simulink model "Fuel_cell"  (R2020b)
settings: Solver=VariableStepAuto  StartTime=0.0  StopTime=10  RelTol=1e-3
undefined symbols (not defined in the file): DiscIntNeverNeededParam, Ion, Lithium, Pbatt, Ts, Vbatt
libraries: powerlib x17, sdl_lib x8, fl_lib x6, nesl_utility x6, simulink x4, AC6DriveInternalModels x3, simulink_extras x2, electricdrivelib x2, powerlib_extras x1, DC6DriveInternalModels x1
(part 1 of 2)
settings Model: Creator=drim  LastModifiedBy=drim

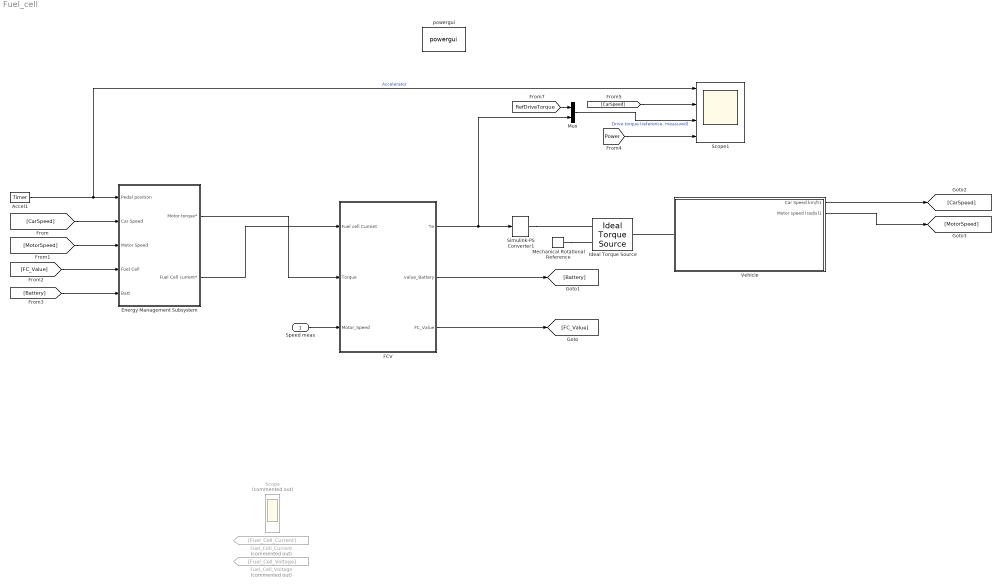
== system Fuel_cell ==
  Speed meas : Inport
  Accel1 : powerlib_extras/Control  Blocks/Timer  t=[0 4 8 12]  e=[0.7 0.25 0.85 -0.7]
      settings: SourceProductBaseCode=PS
  Energy Management Subsystem : Subsystem
      mask init:
      | [X1,X1m,X2,X2m,X3,X4,Y1,Y1m,Y2,Y2m,Y3,Y4,color1,color2]=spsdrivelogo;
      mask Display:
      | patch([X1 X1m],[Y1 Y1m],color1);
      | patch(X3,Y3,color2);
      | plot([X1 X1m X2 X2m X3 X4],[Y1 Y1m Y2 Y2m Y3 Y4]);
  FCV : Subsystem
  Fuel_Cell_Current : Goto  Commented=on  GotoTag=Fuel_Cell_Current
  Fuel_Cell_Voltage : Goto  Commented=on  GotoTag=Fuel_Cell_Voltage
  Ideal Torque Source : fl_lib/Mechanical/Mechanical Sources/Ideal Torque Source
  Mechanical Rotational Reference : fl_lib/Mechanical/Rotational Elements/Mechanical Rotational Reference
  Mux : Mux  Inputs=2
  Scope : Scope  Commented=on  NumInputPorts=3
  Scope1 : Scope  NumInputPorts=4
  Simulink-PS Converter1 : nesl_utility/Simulink-PS Converter  PhysicalDomain=network_engine_domain  SubClassName=ps_input  LeftPortType=input  RightPortType=output  PseudoPeriodic=off  Frequencies=[]  NoiseDistribution=none  NoiseParameters=[]  Unit=1  AffineConversion=off  FilteringAndDerivatives=zero  SimscapeFilterOrder=1  InputFilterTimeConstant=.001  UdotUserProvided=0
  Vehicle : Subsystem
  powergui : powerlib/powergui  Priority=2  SimulationMode=Discrete  SampleTime=Ts  frequency=60  Iterations=50  frequencyindice=0  Pbase=100e6  ErrMax=1e-4  UnitsV=kV  UnitsW=MW  buscounter=0  FunctionMessages=off  echomessages=off  EnableUseOfTLC=off  CurrentSourceSwitches=off  DisableSnubberDevices=off  DisableRonSwitches=off  DisableVfSwitches=off  DisplayEquations=off  AutomaticDiscreteSolvers=off  SolverType=Tustin  Interpol=off  ExternalGateDelay=off  methode=off  Ts=0  x0status=blocks  SPID=off  SwTol=0  HookPort=off  NonlinearTolerance=1e-4  nMaxIteration=100  ContinueOnMaxIteration=off  RestoreLinks=warning  ResistiveCurrentMeasurement=off  Frange=[0:2:500]  Ylog=off  Xlog=on  ShowGrid=off  save=off  variable=ZData  structure=0  ZoomFFT=on  StartTime=0.0  cycles=1  DisplayStyle=1  fundamental=60  FreqAxis=off  MaxFrequency=1000  frequencyindicesteady=1  RmsSteady=1  display=off
  wires:
  Energy Management Subsystem/2(Fuel Cell current*) -> FCV/1(Fuel cell Current)
  Energy Management Subsystem/1(Motor torque*) -> FCV/2("Torque ")
  Speed meas/1 -> FCV/3("Motor_Speed ")
  FCV/1(Te) -> Mux/2, Simulink-PS Converter1/1
  FCV/2(value_Battery) -> [Battery]
  FCV/3(FC_Value) -> [FC_Value]
  Vehicle/1(Car Speed km/h1) -> [CarSpeed]
  Vehicle/2(Motor speed (rad/s)1) -> [MotorSpeed]
  [CarSpeed] -> Energy Management Subsystem/2(Car Speed)
  [MotorSpeed] -> Energy Management Subsystem/3(Motor Speed)
  [FC_Value] -> Energy Management Subsystem/4(Fuel Cell)
  [Battery] -> Energy Management Subsystem/5(Batt)
  Accel1/1 -> Scope1/1, Energy Management Subsystem/1(Pedal position)  "Accelerator"
  [RefDriveTorque] -> Mux/1
  [Power] -> Scope1/4
  Mux/1 -> Scope1/3  "Drive torque (reference, measured)"
  [CarSpeed] -> Scope1/2
  connections:
  Simulink-PS Converter1/RConn1 -- Ideal Torque Source/RConn1
  Mechanical Rotational Reference/LConn1 -- Ideal Torque Source/RConn2
  Vehicle/LConn1 -- Ideal Torque Source/LConn1

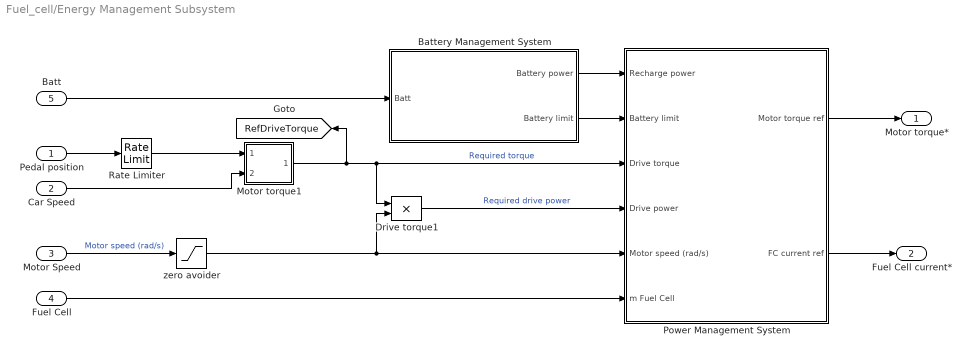
== system Fuel_cell/Energy Management Subsystem ==
  Pedal position : Inport
  Car Speed : Inport  Port=2
  Motor Speed : Inport  Port=3
  Fuel Cell : Inport  Port=4
  Batt : Inport  Port=5
  Battery Management System : Subsystem
      mask init:
      | [X1,X1m,X2,X2m,X3,X4,Y1,Y1m,Y2,Y2m,Y3,Y4,color1,color2]=spsdrivelogo;
      mask Display:
      | patch([X1 X1m],[Y1 Y1m],color1);
      | patch(X3,Y3,color2);
      | plot([X1 X1m X2 X2m X3 X4],[Y1 Y1m Y2 Y2m Y3 Y4]);
  Drive torque1 : Product  Inputs=**  OutDataTypeStr=double
  Motor torque1 : Subsystem
      mask Display: plot([0;1800;2000;2500;3000;3500], [1;1;0.90*1;0.72*1;0.6*1;0.51*1])
  Power Management System : Subsystem
      mask init:
      | [X1,X1m,X2,X2m,X3,X4,Y1,Y1m,Y2,Y2m,Y3,Y4,color1,color2]=spsdrivelogo;
      | power_max = 57000;
      | speed_at_power_max = 5000;
      | speed_max = 6000;
      | [speed,power,torque,p] = drive_enginemodel('MaskGasoline');
      mask Display:
      | patch([X1 X1m],[Y1 Y1m],color1);
      | patch(X3,Y3,color2);
      | plot([X1 X1m X2 X2m X3 X4],[Y1 Y1m Y2 Y2m Y3 Y4]);
  Rate Limiter : RateLimiter  RisingSlewLimit=10  FallingSlewLimit=-10  SampleTimeMode=inherited
  zero avoider : Saturate  UpperLimit=inf  LowerLimit=1
  Motor torque* : Outport
  Fuel Cell current* : Outport  Port=2
  tag scope: RefDriveTorque=global
  wires:
  Motor Speed/1 -> zero avoider/1  "Motor speed (rad/s)"
  Batt/1 -> Battery Management System/1(Batt)
  Pedal position/1 -> Rate Limiter/1
  Fuel Cell/1 -> Power Management System/6(m Fuel Cell)
  Power Management System/1(Motor torque ref) -> Motor torque*/1
  Power Management System/2(FC current ref) -> Fuel Cell current*/1
  Rate Limiter/1 -> Motor torque1/1(Accel)
  Motor torque1/1(torque) -> Drive torque1/1, Power Management System/3(Drive torque), [RefDriveTorque]  "Required torque"
  Drive torque1/1 -> Power Management System/4(Drive power)  "Required drive power"
  Battery Management System/1(Battery power) -> Power Management System/1(Recharge power)
  Car Speed/1 -> Motor torque1/2(N (kmh))
  zero avoider/1 -> Power Management System/5(Motor speed (rad/s)), Drive torque1/2
  Battery Management System/2(Battery limit) -> Power Management System/2(Battery limit)

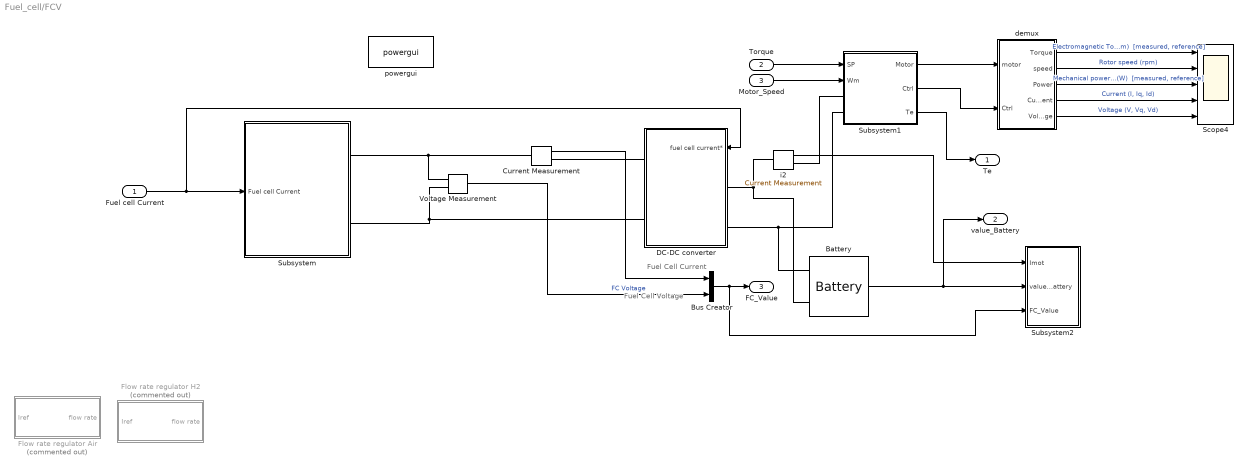
== system Fuel_cell/FCV ==
  note: Fuel Cell Voltage
  note: Fuel Cell Current
  Fuel cell Current : Inport
  "Torque " : Inport  Port=2
  "Motor_Speed " : Inport  Port=3
  Battery : electricdrivelib/Extra Sources/Battery  BatType=Lithium-Ion  ShowTempParam=off  ThermalPreset=no  ShowAgeParam=off  NomV=200  NomQ=5.4  SOC=100  Batt_Tr=30  PresetModel=on  MaxQ=5.4  MinV=150  FullV=232.7974  Dis_rate=2.3478  R=0.37037  Normal_OP=4.8835  expZone="[216.0772     0.2653043]"  current=[6.5 13 32.5]  Units=Time  Tci=20  NomT=20  T2=-30  MaxQ2=4.8  FullV2=7.1  Normal_OP2=5.655  expZone2="[6.58           1]"  Rca=0.6  ti=2000  Dp=0  Neq0=0  Tsim=1e6  Ta1=25  Qeol=5.4*0.9  Reol=0.013333*1.2  Char_age=[2.3478, 3]  Dis_age=[2.3478, 10]  N1=1500  N2=10500  N3=1000  N4=1400  Ta2=45  N5=950
  Bus Creator : BusCreator  Inputs=2
  Current Measurement : powerlib/Measurements/Current Measurement  PhasorSimulation=off  OutputType=Complex  PSBequivalent=0
  DC-DC converter : Subsystem
  Flow rate regulator Air : Subsystem  Commented=on
  Flow rate regulator H2 : Subsystem  Commented=on
  Scope4 : Scope  NumInputPorts=5
  Subsystem : Subsystem
  Subsystem1 : Subsystem
  Subsystem2 : Subsystem
  Voltage Measurement : powerlib/Measurements/Voltage Measurement  PhasorSimulation=off  OutputType=Complex  PSBequivalent=0
  demux : Subsystem
  i2 : powerlib/Measurements/Current Measurement  PhasorSimulation=off  OutputType=Complex  PSBequivalent=0
  powergui : powerlib/powergui  Priority=1  SimulationMode=Discrete  SampleTime=50e-6  frequency=60  Iterations=50  frequencyindice=0  Pbase=100e6  ErrMax=1e-4  UnitsV=kV  UnitsW=MW  buscounter=0  FunctionMessages=off  echomessages=off  EnableUseOfTLC=off  CurrentSourceSwitches=off  DisableSnubberDevices=off  DisableRonSwitches=off  DisableVfSwitches=off  DisplayEquations=off  AutomaticDiscreteSolvers=off  SolverType=Tustin/Backward Euler (TBE)  Interpol=off  ExternalGateDelay=off  methode=off  Ts=100  x0status=blocks  SPID=on  SwTol=0  HookPort=off  NonlinearTolerance=1e-4  nMaxIteration=100  ContinueOnMaxIteration=off  RestoreLinks=warning  ResistiveCurrentMeasurement=off  Frange=[0:2:500]  Ylog=off  Xlog=on  ShowGrid=off  save=off  variable=ZData  structure=0  ZoomFFT=off  StartTime=0.0  cycles=1  DisplayStyle=1  fundamental=60  FreqAxis=off  MaxFrequency=1000  frequencyindicesteady=1  RmsSteady=1  display=off
  Te : Outport
  value_Battery : Outport  Port=2
  FC_Value : Outport  Port=3
  wires:
  Fuel cell Current/1 -> DC-DC converter/1(fuel cell current*), Subsystem/1(Fuel cell Current)
  Bus Creator/1 -> Subsystem2/3(FC_Value), FC_Value/1
  Subsystem1/1(Motor) -> demux/1(motor)
  Battery/1 -> Subsystem2/2(value_Battery), value_Battery/1
  Subsystem1/2(Ctrl) -> demux/2(Ctrl)
  Voltage Measurement/1 -> Bus Creator/2  "FC Voltage"
  "Torque "/1 -> Subsystem1/1(SP)
  Current Measurement/1 -> Bus Creator/1
  "Motor_Speed "/1 -> Subsystem1/2(Wm)
  Subsystem1/3(Te) -> Te/1
  demux/1(Torque) -> Scope4/1  "Electromagnetic Torque (Nm)  [measured, reference]"
  demux/2(speed) -> Scope4/2  "Rotor speed (rpm)"
  demux/3(Power) -> Scope4/3  "Mechanical power (W)  [measured, reference]"
  demux/4(Current) -> Scope4/4  "Current (I, Iq, Id)"
  demux/5(Voltage) -> Scope4/5  "Voltage (V, Vq, Vd)"
  i2/1 -> Subsystem2/1(Imot)
  connections:
  Voltage Measurement/LConn1 -- Current Measurement/LConn1 -- Subsystem/RConn1
  Battery/LConn1 -- i2/LConn1 -- DC-DC converter/LConn1
  Subsystem/RConn2 -- Voltage Measurement/LConn2 -- DC-DC converter/RConn2
  Battery/LConn2 -- Subsystem1/LConn2 -- DC-DC converter/LConn2
  Current Measurement/RConn1 -- DC-DC converter/RConn1
  i2/RConn1 -- Subsystem1/LConn1

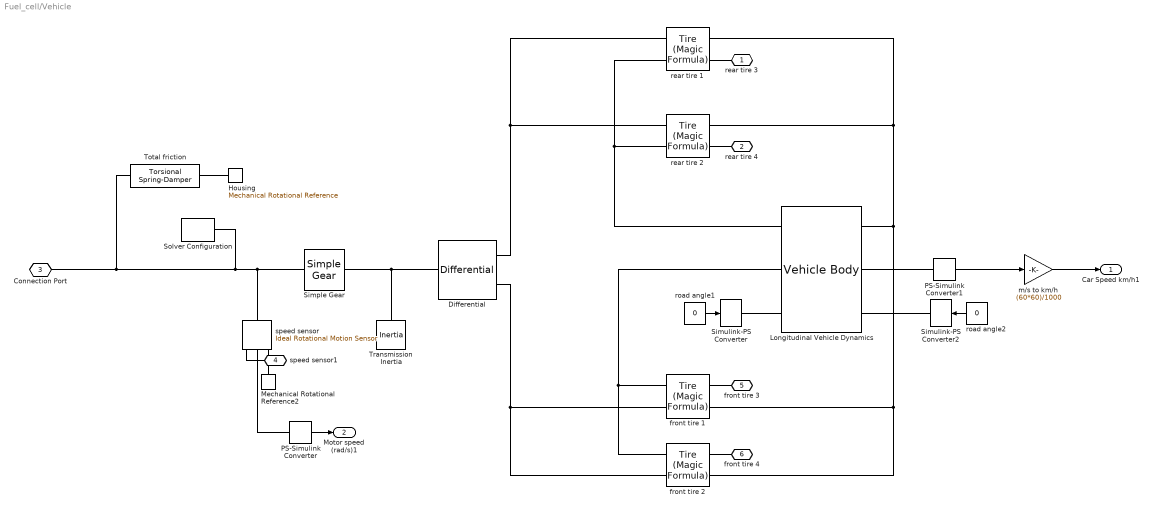
== system Fuel_cell/Vehicle ==
  Differential : sdl_lib/Gears/Differential  driveshaft_location=2  cd_ratio=1  friction_model=1  mu_visc=[ 0 0 ] N*m/(rad/s)  efficiency=[ 0.85 0.92 ]  temperature_TLU=[280, 300, 320] K  efficiency_ss_TLU=[.95, .9, .85]  efficiency_cd_TLU=[.95, .9, .85]  pwr_thr=[.001, .001] W  thermal_mass=50 J/K  T_init=300 K  model_inertia=simscape.enum.onoff.off  carrier_inertia=0.001 kg*m^2  planet_inertia=0.001 kg*m^2
      settings: SourceProductBaseCode=LD
  Housing : fl_lib/Mechanical/Rotational Elements/Mechanical Rotational Reference
  Longitudinal Vehicle Dynamics : sdl_lib/Tires & Vehicles/Vehicle Body  mass=1625 kg  n_w=2  x_f=1.4 m  x_r=1.4 m  y_c=0.5 m  mass_var=simscape.enum.onoff.off  model_pitch=simscape.enum.onoff.off  inertia=4000 kg*m^2  suspension_model=sdl.enum.linearTLU.linear  k_f=1e4 N/m  b_f=1e4 N/(m/s)  k_r=1e4 N/m  b_r=1e4 N/(m/s)  k_f_TLU=[-2000, -1000, 0, 1000, 2000] N  x_f_TLU=[-.4, -.2, 0, .2, .4] m  b_f_TLU=[-200, -100, 0, 100, 200] N  v_f_TLU=[-4, -2, 0, 2, 4] m/s  k_r_TLU=[-2000, -1000, 0, 1000, 2000] N  x_r_TLU=[-.4, -.2, 0, .2, .4] m  b_r_TLU=[-200, -100, 0, 100, 200] N  v_r_TLU=[-4, -2, 0, 2, 4] m/s  interp_method=simscape.enum.interpolation.linear  extrap_method=simscape.enum.extrapolation.linear  model_hardstop=simscape.enum.onoff.off  upper_bound_f=.25 m  lower_bound_f=-.25 m  stop_k_f=1e6 N/m  stop_b_f=150 N/(m/s)  upper_bound_r=.25 m  lower_bound_r=-.25 m  stop_k_r=1e6 N/m  stop_b_r=150 N/(m/s)  initial_pitch=0 rad  initial_pitch_rate=0 rad/s  g=9.81 m/s^2  liftoff_warning=simscape.enum.onoff.off  area=2.711 m^2  Cd=0.26  rho=1.18 kg/m^3  v_specify=on  v_priority=High  v=0 m/s  v_nominal_specify=off  v_nominal_unit=m/s  v_nominal_value=1
  Mechanical Rotational Reference2 : fl_lib/Mechanical/Rotational Elements/Mechanical Rotational Reference
  PS-Simulink Converter : nesl_utility/PS-Simulink Converter  PhysicalDomain=network_engine_domain  SubClassName=ps_output  LeftPortType=input  RightPortType=output  PseudoPeriodic=off  Frequencies=[]  Unit=1  AffineConversion=off
  PS-Simulink Converter1 : nesl_utility/PS-Simulink Converter  PhysicalDomain=network_engine_domain  SubClassName=ps_output  LeftPortType=input  RightPortType=output  PseudoPeriodic=off  Frequencies=[]  Unit=1  AffineConversion=off
  Simple Gear : sdl_lib/Gears/Simple Gear  ratio=7.2  rotation_direction=3-2*(1)  friction_model=1  mu_visc=[ 0 0 ] N*m/(rad/s)  T_noload=0.1 N*m  T_nom=5 N*m  efficiency_nom=0.8  efficiency=0.8  temperature_TLU=[280, 300, 320] K  load_TLU=[1, 5, 10] N*m  efficiency_TLU=[.95, .9, .85]  efficiency_TLU2=[.85, .8, .75; .95, .9, .85; .85, .8, .7]  w_thr=0.01 rad/s  pwr_thr=0.001 W  thermal_mass=50 J/K  enable_faults=simscape.enum.onoff.off  efficiency_fault=0.05  external_fault=simscape.enum.onoff.off  temporal_fault=simscape.enum.onoff.off  fault_time=5 s  fault_angles=pi / 12 rad  report_fault=simscape.enum.assert.action.none  temperature_specify=off  temperature_priority=High  temperature=300 K  temperature_nominal_specify=off  temperature_nominal_unit=K  temperature_nominal_value=1
  Simulink-PS Converter : nesl_utility/Simulink-PS Converter  PhysicalDomain=network_engine_domain  SubClassName=ps_input  LeftPortType=input  RightPortType=output  PseudoPeriodic=off  Frequencies=[]  NoiseDistribution=none  NoiseParameters=[]  Unit=1  AffineConversion=off  FilteringAndDerivatives=zero  SimscapeFilterOrder=1  InputFilterTimeConstant=.001  UdotUserProvided=0
  Simulink-PS Converter2 : nesl_utility/Simulink-PS Converter  PhysicalDomain=network_engine_domain  SubClassName=ps_input  LeftPortType=input  RightPortType=output  PseudoPeriodic=off  Frequencies=[]  NoiseDistribution=none  NoiseParameters=[]  Unit=1  AffineConversion=off  FilteringAndDerivatives=zero  SimscapeFilterOrder=1  InputFilterTimeConstant=.001  UdotUserProvided=0
  Solver Configuration : nesl_utility/Solver Configuration  PhysicalDomain=network_engine_domain  SubClassName=solver  LeftPortType=input  RightPortType=generic  Tones=[]  Harmonics=[]  SimulateNoise=off  Profile=off  UseLocalSampling=off  EnableSwitchedLinearOptims=on  FrequencyDomain=off  UseCCode=off  RelTol=0.001  AbsTol=1e-06  MinStep=1e-09  ToWorkspace=off  RevertToSquareIcSolve=off  NumHomotopyIterations=100  PhasorMode=off  PhasorModeNumHarmonics=1  DoDC=off  ResidualTolerance=1e-5  UseLocalSolver=on  LocalSolverChoice=NE_TRAPEZOIDAL_ADVANCER  LocalSolverSampleTime=Ts  DoFixedCost=off  MaxNonlinIter=3  MaxModeIter=2  ComputeImpulses=off  ImpulseIterations=2  LinearAlgebra=Full  EquationFormulation=NE_TIME_EF  DelaysMemoryBudget=1024  AutomaticFiltering=on  FilteringTimeConstant=0.001  PartitionStorageMethod=AS_NEEDED  PartitionMemoryBudget=1024  PartitionMethod=FAST
  Total friction : sdl_lib/Couplings & Drives/Torsional Spring-Damper  k=0 N*m/rad  mu_visc=0.02 N*m/(rad/s)  trq_coulomb=0 N*m  static_kinetic_ratio=1e9  w_tol=0.001 rad/s  model_hardstop=0  upper_bound=10 deg  lower_bound=-10 deg  k_endstop=1e+6 N*m/rad  D_endstop=10 N*m/(rad/s)  hardstop_model=3  transition=0.001 rad  x0=0 deg
      settings: SourceProductBaseCode=LD  InternalSimscapePortConfiguration="{\"Bottom\":[],\"Left\":[{\"id\":\"R\",\"label\":\"R\",\"type\":\"foundation.mechanical.rotational.rotational\"}],\"Right\":[{\"id\":\"C\",\"label\":\"C\",\"type\":\"foundation.mechanical.rotational.rotational\"}],\"Top\":[]}"
  Transmission Inertia : fl_lib/Mechanical/Rotational Elements/Inertia  inertia=0.5 kg*m^2  num_ports=foundation.enum.numPorts2.one  w_specify=on  w_priority=High  w=0 rad/s  w_nominal_specify=off  w_nominal_unit=rad/s  w_nominal_value=1  t_specify=off  t_priority=High  t=0 N*m  t_nominal_specify=off  t_nominal_unit=N*m  t_nominal_value=1
  front tire 1 : sdl_lib/Tires & Vehicles/Tire (Magic Formula)  parameterization=1  F_z1=3e+3 N  F_x1=3.5e+3 N  kappa1=10  B_m=10  C_m=1.9  D_m=1  E_m=0.97  fz0=4e+3 N  p_Cx=1.685  p_Dx=[ 1.21 -0.037 ]  p_Ex=[ 0.344 0.095 -0.02 0 ]  p_Kx=[ 21.51 -0.163 0.245 ]  p_Hx=[ -0.002 0.002 ]  p_Vx=[ 0 0 ]  v_tr_thr=0.1 m/s  r_e=0.25 m  model_compliance=1  stiffness=1e5 N/m  damping=400 N/(m/s)  model_inertia=1  inertia=0.25 kg*m^2  initial_velocity=0 rad/s  model_resistance=0  resistance_model=1  coeff=0.015  p_tire=250e3 Pa  alpha=-0.003  beta=0.97  coeff_a=84e-4  coeff_b=6.2e-4 s/m  coeff_c=1.6e-4 s^2/m^2  v_thr=1e-3 m/s
  front tire 2 : sdl_lib/Tires & Vehicles/Tire (Magic Formula)  parameterization=1  F_z1=3e+3 N  F_x1=3.5e+3 N  kappa1=10  B_m=10  C_m=1.9  D_m=1  E_m=0.97  fz0=4e+3 N  p_Cx=1.685  p_Dx=[ 1.21 -0.037 ]  p_Ex=[ 0.344 0.095 -0.02 0 ]  p_Kx=[ 21.51 -0.163 0.245 ]  p_Hx=[ -0.002 0.002 ]  p_Vx=[ 0 0 ]  v_tr_thr=0.1 m/s  r_e=0.25 m  model_compliance=1  stiffness=1e5 N/m  damping=400 N/(m/s)  model_inertia=1  inertia=0.25 kg*m^2  initial_velocity=0 rad/s  model_resistance=0  resistance_model=1  coeff=0.015  p_tire=250e3 Pa  alpha=-0.003  beta=0.97  coeff_a=84e-4  coeff_b=6.2e-4 s/m  coeff_c=1.6e-4 s^2/m^2  v_thr=1e-3 m/s
  m/s to km/h : Gain  Gain=(60*60)/1000
  rear tire 1 : sdl_lib/Tires & Vehicles/Tire (Magic Formula)  parameterization=1  F_z1=3e+3 N  F_x1=3.5e+3 N  kappa1=10  B_m=10  C_m=1.9  D_m=1  E_m=0.97  fz0=4e+3 N  p_Cx=1.685  p_Dx=[ 1.21 -0.037 ]  p_Ex=[ 0.344 0.095 -0.02 0 ]  p_Kx=[ 21.51 -0.163 0.245 ]  p_Hx=[ -0.002 0.002 ]  p_Vx=[ 0 0 ]  v_tr_thr=0.1 m/s  r_e=0.25 m  model_compliance=1  stiffness=1e5 N/m  damping=400 N/(m/s)  model_inertia=1  inertia=0.25 kg*m^2  initial_velocity=0 rad/s  model_resistance=0  resistance_model=1  coeff=0.015  p_tire=250e3 Pa  alpha=-0.003  beta=0.97  coeff_a=84e-4  coeff_b=6.2e-4 s/m  coeff_c=1.6e-4 s^2/m^2  v_thr=1e-3 m/s
  rear tire 2 : sdl_lib/Tires & Vehicles/Tire (Magic Formula)  parameterization=1  F_z1=3e+3 N  F_x1=3.5e+3 N  kappa1=10  B_m=10  C_m=1.9  D_m=1  E_m=0.97  fz0=4e+3 N  p_Cx=1.685  p_Dx=[ 1.21 -0.037 ]  p_Ex=[ 0.344 0.095 -0.02 0 ]  p_Kx=[ 21.51 -0.163 0.245 ]  p_Hx=[ -0.002 0.002 ]  p_Vx=[ 0 0 ]  v_tr_thr=0.1 m/s  r_e=0.25 m  model_compliance=1  stiffness=1e5 N/m  damping=400 N/(m/s)  model_inertia=1  inertia=0.25 kg*m^2  initial_velocity=0 rad/s  model_resistance=0  resistance_model=1  coeff=0.015  p_tire=250e3 Pa  alpha=-0.003  beta=0.97  coeff_a=84e-4  coeff_b=6.2e-4 s/m  coeff_c=1.6e-4 s^2/m^2  v_thr=1e-3 m/s
  road angle1 : Constant  Value=0
  road angle2 : Constant  Value=0
  speed sensor : fl_lib/Mechanical/Mechanical Sensors/Ideal Rotational Motion Sensor  wrap_angle=simscape.enum.onoff.off  offset=0 rad
  rear tire 3 : PMIOPort  Side=Right
  rear tire 4 : PMIOPort  Port=2  Side=Right
  Connection Port : PMIOPort  Tag=PMCPort  Port=3  Side=Left
  speed sensor1 : PMIOPort  Port=4  Side=Right
  front tire 3 : PMIOPort  Port=5  Side=Right
  front tire 4 : PMIOPort  Port=6  Side=Right
  Car Speed km/h1 : Outport
  Motor speed (rad/s)1 : Outport  Port=2
  wires:
  m/s to km/h/1 -> Car Speed km/h1/1
  road angle1/1 -> Simulink-PS Converter/1
  PS-Simulink Converter1/1 -> m/s to km/h/1
  road angle2/1 -> Simulink-PS Converter2/1
  PS-Simulink Converter/1 -> Motor speed (rad/s)1/1
  connections:
  Longitudinal Vehicle Dynamics/LConn1 -- front tire 1/RConn2 -- front tire 2/RConn2 -- rear tire 1/RConn2 -- rear tire 2/RConn2
  PS-Simulink Converter1/LConn1 -- Longitudinal Vehicle Dynamics/LConn2
  Simple Gear/RConn1 -- Differential/LConn1 -- Transmission Inertia/LConn1
  front tire 2/LConn2 -- front tire 1/LConn2 -- Differential/RConn1
  Mechanical Rotational Reference2/LConn1 -- speed sensor/RConn1
  Total friction/LConn1 -- Connection Port/RConn1 -- Solver Configuration/RConn1 -- speed sensor/LConn1 -- Simple Gear/LConn1
  front tire 2/LConn1 -- Longitudinal Vehicle Dynamics/RConn2 -- front tire 1/LConn1
  rear tire 1/LConn1 -- Longitudinal Vehicle Dynamics/RConn1 -- rear tire 2/LConn1
  rear tire 1/LConn2 -- rear tire 2/LConn2 -- Differential/RConn2
  speed sensor/RConn3 -- speed sensor1/RConn1
  Simulink-PS Converter/RConn1 -- Longitudinal Vehicle Dynamics/RConn3
  front tire 2/RConn1 -- front tire 4/RConn1
  Simulink-PS Converter2/RConn1 -- Longitudinal Vehicle Dynamics/LConn3
  rear tire 1/RConn1 -- rear tire 3/RConn1
  Housing/LConn1 -- Total friction/RConn1
  PS-Simulink Converter/LConn1 -- speed sensor/RConn2
  front tire 1/RConn1 -- front tire 3/RConn1
  rear tire 2/RConn1 -- rear tire 4/RConn1

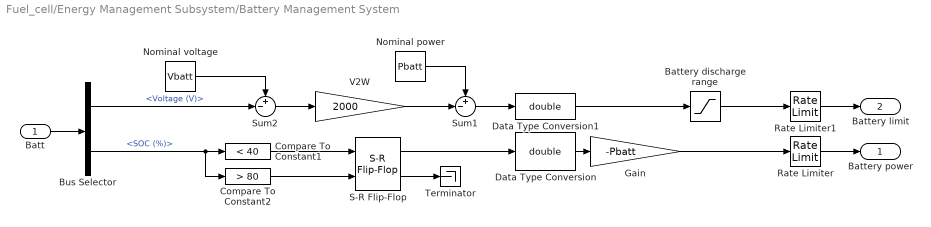
== system Fuel_cell/Energy Management Subsystem/Battery Management System ==
  Batt : Inport
  Battery discharge range : Saturate  UpperLimit=Pbatt  LowerLimit=0
  Bus Selector : BusSelector  OutputSignals=Voltage (V),SOC (%)
  Compare To Constant1 : simulink/Logic and Bit Operations/Compare To Constant  relop=<  const=40  OutDataTypeStr=boolean
  Compare To Constant2 : simulink/Logic and Bit Operations/Compare To Constant  relop=>  const=80  OutDataTypeStr=boolean
  Data Type Conversion : DataTypeConversion  OutDataTypeStr=double  SampleTime=0
  Data Type Conversion1 : DataTypeConversion  OutDataTypeStr=double  SampleTime=0
  Gain : Gain  Gain=-Pbatt
  Nominal power : Constant  Value=Pbatt
  Nominal voltage : Constant  Value=Vbatt
  Rate Limiter : RateLimiter  RisingSlewLimit=Pbatt  FallingSlewLimit=-Pbatt  SampleTimeMode=inherited
  Rate Limiter1 : RateLimiter  RisingSlewLimit=Pbatt*10  FallingSlewLimit=-Pbatt*10  SampleTimeMode=inherited
  S-R Flip-Flop : simulink_extras/Flip Flops/S-R Flip-Flop  initial_condition=0
  Sum1 : Sum  Inputs=+-|
  Sum2 : Sum  Inputs=+-|
  Terminator : Terminator
  V2W : Gain  Gain=2000
  Battery power : Outport
  Battery limit : Outport  Port=2
  wires:
  Batt/1 -> Bus Selector/1
  Gain/1 -> Rate Limiter/1
  S-R Flip-Flop/2 -> Terminator/1
  Bus Selector/2 -> Compare To Constant1/1, Compare To Constant2/1  "<SOC (%)>"
  Data Type Conversion/1 -> Gain/1
  Compare To Constant1/1 -> S-R Flip-Flop/1
  Compare To Constant2/1 -> S-R Flip-Flop/2
  S-R Flip-Flop/1 -> Data Type Conversion/1
  Sum2/1 -> V2W/1
  V2W/1 -> Sum1/2
  Nominal power/1 -> Sum1/1
  Sum1/1 -> Data Type Conversion1/1
  Data Type Conversion1/1 -> Battery discharge range/1
  Battery discharge range/1 -> Rate Limiter1/1
  Bus Selector/1 -> Sum2/2  "<Voltage (V)>"
  Nominal voltage/1 -> Sum2/1
  Rate Limiter1/1 -> Battery limit/1
  Rate Limiter/1 -> Battery power/1

== system Fuel_cell/Energy Management Subsystem/Motor torque1 ==
  Accel : Inport
  N (kmh) : Inport  Port=2
  Abs1 : Abs  SaturateOnIntegerOverflow=on
  Abs2 : Abs  SaturateOnIntegerOverflow=on
  MinMax : MinMax  Inputs=2
  Product : Product  RndMeth=Zero
  Sign : Signum
  Torque vs speed profile : Lookup  InputValues=[0 20 38 60 80 100 120 135 160]  Table=[256 256 256 203 152 122 101 90.5 61]
  rad/s to rpm1 : Gain  Gain=256
  torque : Outport
  wires:
  N (kmh)/1 -> Abs1/1
  Accel/1 -> Abs2/1, Sign/1
  rad/s to rpm1/1 -> MinMax/2
  Torque vs speed profile/1 -> MinMax/1
  Abs1/1 -> Torque vs speed profile/1
  Abs2/1 -> rad/s to rpm1/1
  MinMax/1 -> Product/1
  Sign/1 -> Product/2
  Product/1 -> torque/1

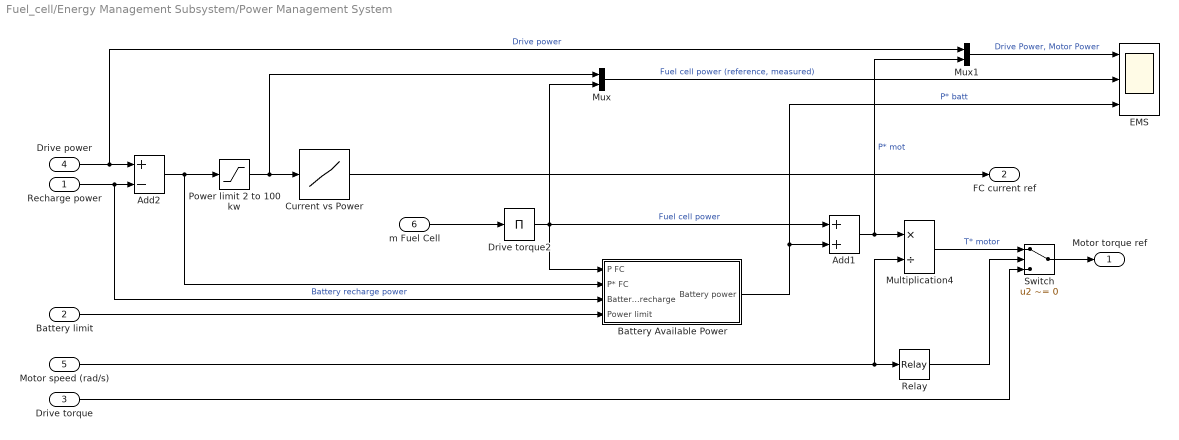
== system Fuel_cell/Energy Management Subsystem/Power Management System ==
  Recharge power : Inport
  Battery limit : Inport  Port=2
  Drive torque : Inport  Port=3
  Drive power : Inport  Port=4
  Motor speed (rad/s) : Inport  Port=5
  m Fuel Cell : Inport  Port=6
  Add1 : Sum
  Add2 : Sum  Inputs=+-
  Battery Available Power : Subsystem
  Current vs Power : Lookup  InputValues=[0,159.95,479.63,795.54,1098.9,1397.7,1691.6,1982,2269.3,2554.2,2837,3117.8,3396.8,3674.2,3950.2,4224.8,4498.1,4770.1,5041,5310.8,5579.6,5847.4,6114.2,6380,6645,6909.1,7172.4,7434.9,7696.5,7957.4,8217.6,8477,8735.7,8993.8,9251.1,9507.8,9763.8,10019,10274,10528,10782,11034,11287,11538,11790,12040,12290,12540,12789,13037,13285,13533,13779,14026,14272,14517,14762,15006,15250,15494,15737,15979,16221,16463,16704,16945,17185,17425,17664,17903,18141,18379,18617,18854,19091,19327,19563,19799,20034,20269,20503,20737,20970,21204,21436,21669,21901,22132,22363,22594,22825,23055,23284,23514,23743,23971,24199,24427,24655,24882,25108,25335,25561,25786,26012,26237,26461,26686,26909,27133,27356,27579,27802,28024,28246,28467,28688,28909,29130,29350,29570,29789,30008,30227,30446,30664,30882,31099,31317,31534,31750,31967,32182,32398,32613,32828,33043,33258,33472,33685,33899,34112,34325,34537,34750,34962,35173,35385,35596,35806,36017,36227,36437,36646,36855,37064,37273,37481,37689,37897,38105,38312,38519,38725,38932,39138,39343,39549,39754,39959,40163,40368,40572,40775,40979,41182,41385,41588,41790,41992,42194,42395,42596,42797,42998,43198,43399,43598,43798,43997,44196,44395,44594,44792,44990,45188,45385,45582,45779,45976,46172,46368,46564,46760,46955,47150,47345,47539,47733,47927,48121,48315,48508,48701,48894,49086,49278,49470,49662,49853,50044,50235,50426,50616,50807,50996,51186,51375,51565,51754,51942,52131,52319,52507,52694,52882,53069,53256,53442,53629,53815,54001,54187,54372,54557,54742,54927,55111,55296,55480,55663,55847,56030,56213,56396,56578,56761,56943,57125,57306,57487,57669,57849,58030,58210,58391,58571,58750,58930,59109,59288,59467,59645,59824,60002,60179,60357,60534,60712,60888,61065,61242,61418,61594,61770,61945,62120,62296,62470,62645,62819,62994,63168,63341,63515,63688,63861,64034,64207,64379,64551,64723,64895,65066,65238,65409,65580,65750,65921,66091,66261,66430,66600,66769,66938,67107,67276,67444,67612,67780,67948,68116,68283,68450,68617,68784,68950,69117,69283,69449,69614,69780,69945,70110,70275,70439,70604,70768,70932,71095,71259,71422,71585,71748,71911,72073,72236,72398,72560,72721,72883,73044,73205,73366,73526,73687,73847,74007,74167,74326,74486,74645,74804,74963,75121,75280,75438,75596,75753,75911,76068,76225,76382,76539,76696,76852,77008,77164,77320,77475,77631,77786,77941,78096,78250,78404,78559,78713,78866,79020,79173,79326,79479,79632,79785,79937,80089,80241,80393,80545,80696,80847,80998,81149,81300,81450,81600,81751,81900,82050,82200,82349,82498,82647,82796,82944,83092,83241,83389,83536,83684,83831,83978,84125,84272,84419,84565,84712,84858,85004,85149,85295,85440,85585,85730,85875,86020,86164,86308,86452,86596,86740,86883,87026,87169,87312,87455,87598,87740,87882,88024,88166,88308,88449,88590,88731,88872,89013,89154,89294,89434,89574,89714,89854,89993,90132,90271,90410,90549,90688,90826,90964,91102,91240,91378,91515,91653,91790,91927,92064,92200,92337,92473,92609,92745,92881,93016,93152,93287,93422,93557,93691,93826,93960,94094,94228,94362,94496,94629,94763,94896,95029,95162,95294,95427,95559,95691,95823,95955,96086,96218,96349,96480,96611,96742,96872,97003,97133,97263,97393,97523,97652,97782,97911,98040,98169,98297,98426,98554,98683,98811,98939,99066,99194,99321,99448,99575,99702,99829,99956,1.0002e+005]  Table=[0,0.39993,1.1997,1.9991,2.7965,3.5871,4.3694,5.1459,5.9178,6.6861,7.4512,8.2135,8.9735,9.7311,10.487,11.241,11.993,12.743,13.492,14.239,14.985,15.73,16.474,17.216,17.957,18.697,19.436,20.174,20.911,21.647,22.382,23.116,23.849,24.581,25.313,26.043,26.773,27.502,28.23,28.958,29.684,30.41,31.136,31.86,32.584,33.307,34.029,34.751,35.472,36.193,36.912,37.632,38.35,39.068,39.785,40.502,41.218,41.934,42.649,43.363,44.077,44.79,45.503,46.215,46.926,47.637,48.348,49.058,49.767,50.476,51.184,51.892,52.599,53.306,54.013,54.718,55.424,56.129,56.833,57.537,58.24,58.943,59.646,60.348,61.049,61.75,62.451,63.151,63.85,64.55,65.248,65.947,66.645,67.342,68.039,68.735,69.432,70.127,70.822,71.517,72.212,72.906,73.599,74.292,74.985,75.677,76.369,77.06,77.751,78.442,79.132,79.822,80.511,81.2,81.889,82.577,83.265,83.952,84.639,85.326,86.012,86.698,87.383,88.068,88.753,89.437,90.121,90.805,91.488,92.17,92.853,93.535,94.216,94.898,95.578,96.259,96.939,97.619,98.298,98.977,99.656,100.33,101.01,101.69,102.37,103.04,103.72,104.4,105.07,105.75,106.42,107.1,107.77,108.45,109.12,109.79,110.47,111.14,111.81,112.48,113.15,113.82,114.5,115.17,115.84,116.51,117.18,117.84,118.51,119.18,119.85,120.52,121.18,121.85,122.52,123.19,123.85,124.52,125.18,125.85,126.51,127.18,127.84,128.5,129.17,129.83,130.49,131.16,131.82,132.48,133.14,133.8,134.46,135.12,135.78,136.44,137.1,137.76,138.42,139.08,139.74,140.4,141.05,141.71,142.37,143.03,143.68,144.34,144.99,145.65,146.3,146.96,147.61,148.27,148.92,149.58,150.23,150.88,151.53,152.19,152.84,153.49,154.14,154.79,155.44,156.09,156.74,157.39,158.04,158.69,159.34,159.99,160.64,161.29,161.94,162.58,163.23,163.88,164.52,165.17,165.82,166.46,167.11,167.75,168.4,169.04,169.69,170.33,170.97,171.62,172.26,172.9,173.55,174.19,174.83,175.47,176.11,176.75,177.39,178.03,178.67,179.31,179.95,180.59,181.23,181.87,182.51,183.15,183.78,184.42,185.06,185.7,186.33,186.97,187.61,188.24,188.88,189.51,190.15,190.78,191.42,192.05,192.68,193.32,193.95,194.58,195.22,195.85,196.48,197.11,197.75,198.38,199.01,199.64,200.27,200.9,201.53,202.16,202.79,203.42,204.05,204.67,205.3,205.93,206.56,207.19,207.81,208.44,209.07,209.69,210.32,210.94,211.57,212.2,212.82,213.45,214.07,214.69,215.32,215.94,216.56,217.19,217.81,218.43,219.06,219.68,220.3,220.92,221.54,222.16,222.78,223.4,224.02,224.64,225.26,225.88,226.5,227.12,227.74,228.36,228.98,229.59,230.21,230.83,231.45,232.06,232.68,233.29,233.91,234.53,235.14,235.76,236.37,236.99,237.6,238.21,238.83,239.44,240.06,240.67,241.28,241.89,242.51,243.12,243.73,244.34,244.95,245.56,246.17,246.78,247.39,248,248.61,249.22,249.83,250.44,251.05,251.66,252.27,252.87,253.48,254.09,254.7,255.3,255.91,256.52,257.12,257.73,258.33,258.94,259.54,260.15,260.75,261.36,261.96,262.57,263.17,263.77,264.38,264.98,265.58,266.18,266.79,267.39,267.99,268.59,269.19,269.79,270.39,270.99,271.59,272.19,272.79,273.39,273.99,274.59,275.19,275.79,276.38,276.98,277.58,278.18,278.77,279.37,279.97,280.56,281.16,281.76,282.35,282.95,283.54,284.14,284.73,285.33,285.92,286.51,287.11,287.7,288.29,288.89,289.48,290.07,290.66,291.26,291.85,292.44,293.03,293.62,294.21,294.8,295.39,295.98,296.57,297.16,297.75,298.34,298.93,299.52,300.11,300.69,301.28,301.87,302.46,303.04,303.63,304.22,304.8,305.39,305.98,306.56,307.15,307.73,308.32,308.9,309.49,310.07,310.65,311.24,311.82,312.41,312.99,313.57,314.15,314.74,315.32,315.9,316.48,317.06,317.64,318.23,318.81,319.39,319.97,320.55,321.13,321.71,322.29,322.86,323.44,324.02,324.6,325.18,325.76,326.33,326.91,327.49,328.07,328.64,329.22,329.79,330.37,330.95,331.52,332.1,332.67,333.25,333.82,334.4,334.97,335.54,336.12,336.69,337.26,337.84,338.41,338.98,339.56,340.13,340.7,341.27,341.84,342.41,342.98,343.56,344.13,344.7,345.27,345.84,346.41,346.98,347.54]
  Drive torque2 : Product  Inputs=*  OutDataTypeStr=double
  EMS : Scope  NumInputPorts=3
  Multiplication4 : Product  Inputs=*/
  Mux : Mux  Inputs=2
  Mux1 : Mux  Inputs=2
  Power limit 2 to 100 kw : Saturate  UpperLimit=100e3  LowerLimit=2e3
  Relay : Relay  OnSwitchValue=300/30*pi  OffSwitchValue=200/30*pi
  Switch : Switch  Criteria=u2 ~= 0
  Motor torque ref : Outport
  FC current ref : Outport  Port=2
  wires:
  Motor speed (rad/s)/1 -> Relay/1, Multiplication4/2
  Drive torque2/1 -> Add1/1, Mux/2, Battery Available Power/1(P FC)  "Fuel cell power"
  Add1/1 -> Multiplication4/1, Mux1/2  "P* mot"
  Drive power/1 -> Add2/1, Mux1/1  "Drive power"
  Add2/1 -> Power limit 2 to 100 kw/1, Battery Available Power/2(P* FC)
  Battery Available Power/1(Battery power) -> Add1/2, EMS/3  "P* batt"
  Current vs Power/1 -> FC current ref/1
  Recharge power/1 -> Add2/2, Battery Available Power/3(Battery recharge)  "Battery recharge power"
  Battery limit/1 -> Battery Available Power/4(Power limit)
  m Fuel Cell/1 -> Drive torque2/1
  Mux/1 -> EMS/2  "Fuel cell power (reference, measured)"
  Power limit 2 to 100 kw/1 -> Current vs Power/1, Mux/1
  Relay/1 -> Switch/2
  Multiplication4/1 -> Switch/1  "T* motor"
  Switch/1 -> Motor torque ref/1
  Drive torque/1 -> Switch/3
  Mux1/1 -> EMS/1  "Drive Power, Motor Power"

== system Fuel_cell/FCV/DC-DC converter ==
  fuel cell current* : Inport
  Bus DC controller : Subsystem
  DC/DC converter : Subsystem
  +Vfc : PMIOPort  Tag=PMCPort  Side=Right
  - Vfc : PMIOPort  Tag=PMCPort  Port=2  Side=Right
  + Vdc : PMIOPort  Tag=PMCPort  Port=3  Side=Left
  - Vdc : PMIOPort  Tag=PMCPort  Port=4  Side=Left
  wires:
  DC/DC converter/1(ifc) -> Bus DC controller/2(ifc)
  Bus DC controller/1(Duty cycle) -> DC/DC converter/1(Duty Cycle)
  fuel cell current*/1 -> Bus DC controller/1(iref)
  connections:
  + Vdc/RConn1 -- DC/DC converter/RConn1
  +Vfc/RConn1 -- DC/DC converter/LConn1
  - Vfc/RConn1 -- DC/DC converter/LConn2
  - Vdc/RConn1 -- DC/DC converter/RConn2

== system Fuel_cell/FCV/Flow rate regulator Air ==
  Iref : Inport
  Compressor response : TransferFcn  Denominator=[1/3 1]
  Fcn1 : Fcn  Expr=60000*8.3145*(273+95)*400*u(1)/(4*96485*(3*101325)*0.5057*.21)
  Saturation : Saturate  UpperLimit=inf  LowerLimit=60
  flow rate : Outport
  wires:
  Iref/1 -> Fcn1/1
  Saturation/1 -> flow rate/1
  Fcn1/1 -> Compressor response/1
  Compressor response/1 -> Saturation/1

== system Fuel_cell/FCV/Flow rate regulator H2 ==
  Iref : Inport
  Fcn1 : Fcn  Expr=60000*8.3145*(273+95)*400*u(1)/(2*96485*(3*101325)*0.919*.9995)
  Saturation : Saturate  UpperLimit=inf  LowerLimit=1
  flow rate : Outport
  wires:
  Fcn1/1 -> Saturation/1
  Saturation/1 -> flow rate/1
  Iref/1 -> Fcn1/1

== system Fuel_cell/FCV/Subsystem ==
  Fuel cell Current : Inport
  Bus Selector : BusSelector  OutputSignals=Current
  Fcn1 : Fcn  Expr=60000*8.3145*(273+95)*400*u(1)/(2*96485*(3*101325)*0.919*.9995)
  Fcn2 : Fcn  Expr=60000*8.3145*(273+95)*400*u(1)/(4*96485*(3*101325)*0.5057*.21)
  Fuel Cell Stack : electricdrivelib/Extra Sources/Fuel Cell Stack  PresetModel=PEMFC - 6 kW - 45 Vdc  FcType=Proton Exchange Membrane (PEM)  Detailed=Detailed  Eoc=[65,63]  NomVI=[133.3,45]  EndVI=[225,37]  Nc=65  n=55  TOp=65  AirFr=300  SuppPress=[1.5,1]  Comp=[99.95,21,1]  SignX=off  SignY=off  FlowRateH2=on  FlowRateAir=on  SystemTemp=off  SystemPH2=off  SystemPAir=off  FCDyn=on  FC_tau=2  Peak_O2=80  V_Under=10
      settings: SourceProductBaseCode=PS
  MinMax : MinMax  Function=max  Inputs=2
  +Vfc : PMIOPort  Side=Right
  -Vfc : PMIOPort  Port=2  Side=Right
  wires:
  MinMax/1 -> Fcn2/1, Fcn1/1
  Bus Selector/1 -> MinMax/1  "<Current>"
  Fuel cell Current/1 -> MinMax/2
  Fcn1/1 -> Fuel Cell Stack/1
  Fcn2/1 -> Fuel Cell Stack/2
  Fuel Cell Stack/1 -> Bus Selector/1
  connections:
  +Vfc/RConn1 -- Fuel Cell Stack/RConn1
  -Vfc/RConn1 -- Fuel Cell Stack/RConn2

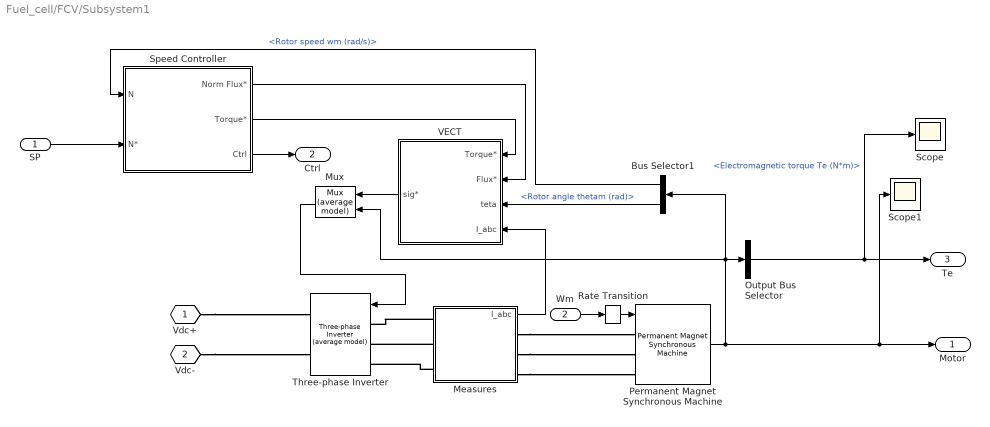
== system Fuel_cell/FCV/Subsystem1 ==
  SP : Inport
  Wm : Inport  Port=2
  Bus Selector1 : BusSelector  OutputSignals=Rotor speed wm (rad/s),Rotor angle thetam (rad)
  Measures : Subsystem
  Mux : AC6DriveInternalModels/Mux (average model)  SystemSampleTime=-1  VariantActivationTime=update diagram  Latency=0  AutoFrameSizeCalculation=off
      settings: SourceProductBaseCode=PS
  Output Bus Selector : BusSelector  OutputSignals=Electromagnetic torque Te (N*m)
  Permanent Magnet Synchronous Machine : powerlib/Machines/Permanent Magnet Synchronous Machine  NbPhases=3  FluxDistribution=Sinusoidal  RotorType=Salient-pole  MechanicalLoad=Speed w  PresetModel=No  ShowDetailedParameters=on  MeasurementBus=off  Resistance=18.7  Inductance=0  dqInductances=[0.02547 0.02816]  La=0.000835  MachineConstant=Flux linkage established by magnets (V.s)  Flux=0.1716  VoltageCst=62.2496  TorqueCst=0.5148  Flat=0  Mechanical=[2.26e-05 1.349e-05 2 0]  PolePairs=2  InitialConditions=[0,0, 0,0]  InitialConditions5ph=[0 0 0 0 0 0]  RefAngle=90 degrees behind phase A axis (modified Park)  IterativeDiscreteModel=Trapezoidal non iterative  TsBlock=-1  TsPowergui=0
      settings: AttributesFormatString=\n
  Rate Transition : RateTransition  OutPortSampleTime=Ts
  Scope : Scope
  Scope1 : Scope
  Speed Controller : Subsystem  mask(Speed controller){SwK=Torque regulation, ramp=[-1000,1000]*10, kp=5, ki=100, fc=100, ctrl_sat=[-256 256], Tsc=120e-6}
      mask prompts: SwK "Regulation type"; ramp "Speed reference ramp (rpm/s) [deceleration,acceleration]"; kp "Proportional gain"; ki "Integral gain"; fc "Speed measurement - low-pass filter cutoff frequency (Hz)"; ctrl_sat "Controller output torque saturation (N.m) [negative,positive]"; Tsc "Controller sampling time (s)"
      mask help: This block implements a PI speed regulator.
      mask init:
      | [X1,X1m,X2,X2m,X3,X4,Y1,Y1m,Y2,Y2m,Y3,Y4,color1,color2]=spsdrivelogo;
      | if SwK == 1
      |     set_param(gcb,'MaskVisibilities',{'on','on','on','on','on','on','on'})
      | else
      |     set_param(gcb,'MaskVisibilities',{'on','off','off','off','off','on','on'})
      | end
      mask TypeOptions SwK: Speed regulation | Torque regulation
      mask Display:
      | patch([X1 X1m],[Y1 Y1m],color1);
      | patch(X3,Y3,color2);
      | plot([X1 X1m X2 X2m X3 X4],[Y1 Y1m Y2 Y2m Y3 Y4]);
  Three-phase Inverter : AC6DriveInternalModels/Three-phase Inverter (average model)  Arms=3  SnubberResistance=5000  SnubberCapacitance=inf  Device=IGBT / Diodes  Ron=1e-3  Lon=0  ForwardVoltages=[0.8,0.8]  ForwardVoltage=0  GTOparameters=[0,0]  IGBTparameters=[1e-6,2e-6]  Measurements=All voltages and currents  converterType=Inverter  SourceFrequency=60  dqInductances="[0.00017415845761   0.00029268882377]"  Flux=0.07111510954334  Resistance=0.0083  p=4
      settings: SourceProductBaseCode=PS
  VECT : Subsystem  mask(VECT){nb_p=4, dqInductances=[0.00017415845761   0.00029268882377], lambda=0.07111510954334, freq_max=20e3, Ts_vect=60e-6, h=0.1}
      mask prompts: nb_p "Motor pairs of poles"; dqInductances "Inductances [ Ld(H) Lq(H) ]:"; lambda "Flux induced by magnets (Wb)"; freq_max "Maximum switching frequency (Hz)"; Ts_vect "Sampling time (s)"; h "Current hysteresis bandwidth (A)"
      mask help: This block implements a vector controller.
      mask init:
      | [X1,X1m,X2,X2m,X3,X4,Y1,Y1m,Y2,Y2m,Y3,Y4,color1,color2]=spsdrivelogo;
      | ib = lambda/(dqInductances(2)-dqInductances(1));
      | Teb = 3/2*nb_p*lambda*ib;
      mask Display:
      | patch([X1 X1m],[Y1 Y1m],color1);
      | patch(X3,Y3,color2);
      | plot([X1 X1m X2 X2m X3 X4],[Y1 Y1m Y2 Y2m Y3 Y4]);
  Vdc+ : PMIOPort  Tag=PMCPort  Side=Left
  Vdc- : PMIOPort  Tag=PMCPort  Port=2  Side=Left
  Motor : Outport
  Ctrl : Outport  Port=2
  Te : Outport  Port=3
  wires:
  Bus Selector1/2 -> VECT/3(teta)  "<Rotor angle thetam (rad)>"
  Speed Controller/3(Ctrl) -> Ctrl/1
  Output Bus Selector/1 -> Scope/1, Te/1  "<Electromagnetic torque Te (N*m)>"
  Mux/1 -> Three-phase Inverter/1
  Rate Transition/1 -> Permanent Magnet Synchronous Machine/1
  SP/1 -> Speed Controller/2(N*)
  Wm/1 -> Rate Transition/1
  VECT/1(sig*) -> Mux/1
  Speed Controller/1(Norm Flux*) -> VECT/2(Flux*)
  Speed Controller/2(Torque*) -> VECT/1(Torque*)
  Permanent Magnet Synchronous Machine/1 -> Scope1/1, Motor/1, Mux/2, Output Bus Selector/1, Bus Selector1/1
  Measures/1(I_abc) -> VECT/4(I_abc)
  Bus Selector1/1 -> Speed Controller/1(N)  "<Rotor speed wm (rad/s)>"
  connections:
  Vdc-/RConn1 -- Three-phase Inverter/RConn2
  Measures/LConn2 -- Three-phase Inverter/LConn2
  Vdc+/RConn1 -- Three-phase Inverter/RConn1
  Measures/RConn2 -- Permanent Magnet Synchronous Machine/LConn2
  Measures/LConn3 -- Three-phase Inverter/LConn3
  Measures/RConn1 -- Permanent Magnet Synchronous Machine/LConn1
  Measures/RConn3 -- Permanent Magnet Synchronous Machine/LConn3
  Measures/LConn1 -- Three-phase Inverter/LConn1

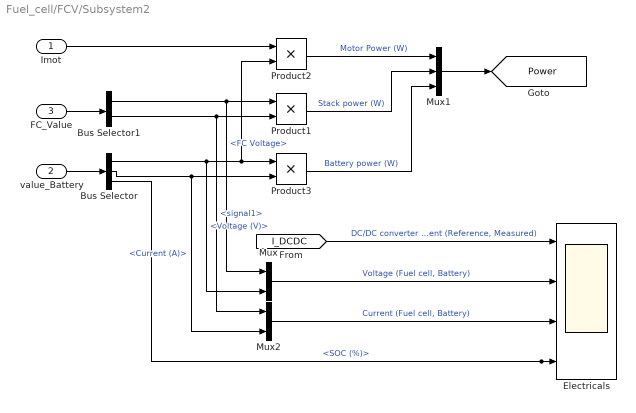
== system Fuel_cell/FCV/Subsystem2 ==
  Imot : Inport
  value_Battery : Inport  Port=2
  FC_Value : Inport  Port=3
  Bus Selector : BusSelector  OutputSignals=Voltage (V),Current (A),SOC (%)
  Bus Selector1 : BusSelector  OutputSignals=FC Voltage,signal1
  Electricals : Scope  NumInputPorts=4
  Mux : Mux  Inputs=2
  Mux1 : Mux  Inputs=3
  Mux2 : Mux  Inputs=2
  Product1 : Product  RndMeth=Zero
  Product2 : Product  RndMeth=Zero
  Product3 : Product  RndMeth=Zero
  tag scope: Power=global
  wires:
  Mux/1 -> Electricals/2  "Voltage (Fuel cell, Battery)"
  Product1/1 -> Mux1/2  "Stack power (W)"
  Imot/1 -> Product2/1
  Bus Selector/1 -> Mux/2, Product3/1, Product2/2  "<Voltage (V)>"
  FC_Value/1 -> Bus Selector1/1
  Bus Selector/3 -> Electricals/4  "<SOC (%)>"
  Bus Selector1/1 -> Product1/1, Mux/1  "<FC Voltage>"
  Bus Selector1/2 -> Product1/2, Mux2/1  "<signal1>"
  Mux1/1 -> [Power]
  Bus Selector/2 -> Product3/2, Mux2/2  "<Current (A)>"
  Product2/1 -> Mux1/1  "Motor Power (W)"
  value_Battery/1 -> Bus Selector/1
  Mux2/1 -> Electricals/3  "Current (Fuel cell, Battery)"
  [I_DCDC] -> Electricals/1  "DC/DC converter current (Reference, Measured)"
  Product3/1 -> Mux1/3  "Battery power (W)"

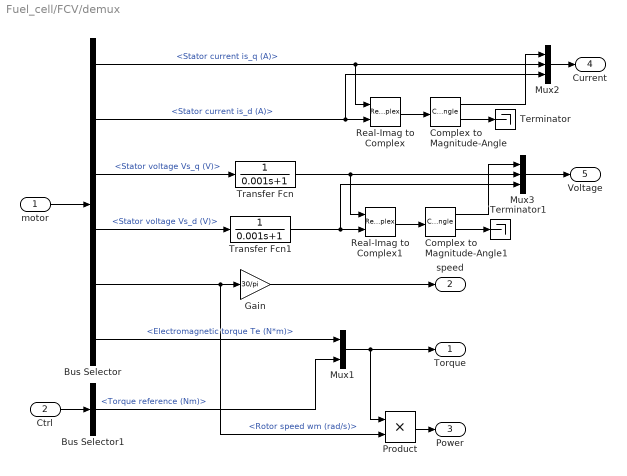
== system Fuel_cell/FCV/demux ==
  motor : Inport
  Ctrl : Inport  Port=2
  Bus Selector : BusSelector  OutputSignals=Stator current is_q (A),Stator current is_d (A),Stator voltage Vs_q (V),Stator voltage Vs_d (V),Rotor speed wm (rad/s),Electromagnetic torque Te (N*m)
  Bus Selector1 : BusSelector  OutputSignals=Torque reference (Nm)
  Complex to Magnitude-Angle : ComplexToMagnitudeAngle
  Complex to Magnitude-Angle1 : ComplexToMagnitudeAngle
  Gain : Gain  Gain=30/pi  SaturateOnIntegerOverflow=on  OutDataTypeStr=Inherit: Same as input  ParamDataTypeStr=Inherit: Same as input
  Mux1 : Mux  Inputs=2
  Mux2 : Mux  Inputs=3
  Mux3 : Mux  Inputs=3
  Product : Product  RndMeth=Zero
  Real-Imag to Complex : RealImagToComplex
  Real-Imag to Complex1 : RealImagToComplex
  Terminator : Terminator
  Terminator1 : Terminator
  Transfer Fcn : TransferFcn  Denominator=[0.001 1]
  Transfer Fcn1 : TransferFcn  Denominator=[0.001 1]
  Torque : Outport
  speed : Outport  Port=2
  Power : Outport  Port=3
  Current : Outport  Port=4
  Voltage : Outport  Port=5
  wires:
  Bus Selector/5 -> Gain/1, Product/2  "<Rotor speed wm (rad/s)>"
  Ctrl/1 -> Bus Selector1/1
  Gain/1 -> speed/1
  Mux1/1 -> Torque/1, Product/1
  motor/1 -> Bus Selector/1
  Mux2/1 -> Current/1
  Product/1 -> Power/1
  Bus Selector/2 -> Real-Imag to Complex/2, Mux2/3  "<Stator current is_d (A)>"
  Bus Selector/1 -> Real-Imag to Complex/1, Mux2/2  "<Stator current is_q (A)>"
  Real-Imag to Complex/1 -> Complex to Magnitude-Angle/1
  Complex to Magnitude-Angle/2 -> Terminator/1
  Complex to Magnitude-Angle/1 -> Mux2/1
  Mux3/1 -> Voltage/1
  Bus Selector/4 -> Transfer Fcn1/1  "<Stator voltage Vs_d (V)>"
  Bus Selector/3 -> Transfer Fcn/1  "<Stator voltage Vs_q (V)>"
  Real-Imag to Complex1/1 -> Complex to Magnitude-Angle1/1
  Complex to Magnitude-Angle1/2 -> Terminator1/1
  Complex to Magnitude-Angle1/1 -> Mux3/1
  Transfer Fcn/1 -> Mux3/2, Real-Imag to Complex1/1
  Transfer Fcn1/1 -> Mux3/3, Real-Imag to Complex1/2
  Bus Selector/6 -> Mux1/1  "<Electromagnetic torque Te (N*m)>"
  Bus Selector1/1 -> Mux1/2  "<Torque reference (Nm)>"

== system Fuel_cell/Energy Management Subsystem/Power Management System/Battery Available Power ==
  P FC : Inport
  P* FC : Inport  Port=2
  Battery recharge : Inport  Port=3
  Power limit : Inport  Port=4
  Add2 : Sum  Inputs=-+
  Compare To Zero : simulink/Logic and Bit Operations/Compare To Zero  relop=~=  OutDataTypeStr=boolean
  Gain : Gain  Gain=-1
  Rate Limiter : RateLimiter  RisingSlewLimit=Pbatt  FallingSlewLimit=-Pbatt  SampleTimeMode=inherited
  Saturation Dynamic : simulink/Discontinuities/Saturation Dynamic  OutMin=[]  OutMax=[]  OutDataTypeStr=Inherit: Same as second input  OutDataType=sfix(16)  OutScaling=2^-10  DoSatur=off
  Switch1 : Switch  Criteria=u2 ~= 0
  Switch2 : Switch  Criteria=u2 ~= 0
  Battery power : Outport
  wires:
  Battery recharge/1 -> Switch1/1, Compare To Zero/1
  Compare To Zero/1 -> Switch1/2, Switch2/2
  P FC/1 -> Add2/1
  Saturation Dynamic/1 -> Battery power/1
  P* FC/1 -> Add2/2
  Add2/1 -> Switch1/3, Switch2/3  "P batt"
  Power limit/1 -> Gain/1, Saturation Dynamic/1
  Gain/1 -> Saturation Dynamic/3
  Switch1/1 -> Rate Limiter/1
  Rate Limiter/1 -> Switch2/1
  Switch2/1 -> Saturation Dynamic/2

== system Fuel_cell/FCV/DC-DC converter/Bus DC controller ==
  iref : Inport
  ifc : Inport  Port=2
  Current controller DISCRETE1 : Subsystem  mask(PI controller){Kp=0.0005, Ki=0.1, Ts=6e-5}
      mask prompts: Kp "Proportional gain (Kp)"; Ki "Integral gain (Ki)"; Ts "Sample time (s) :"
      mask help: Proportional-Integral Speed Controller
      mask Display: plot(0,0,100,100,[35,35,65],[70,30,30],[35,65],[45,60])
  Duty Cycles : Subsystem
  Fuel cell current limit : TransferFcn  Denominator=[1.5/3 1]
  Mux : Mux  Inputs=2
  Transfer Fcn (with initial outputs)2 : simulink_extras/Additional Linear/Transfer Fcn (with initial outputs)  N=[1]  D="[.0001  1]"  Y0=0  U0=0
  Zero-Order Hold1 : ZeroOrderHold  SampleTime=Ts
  Duty cycle : Outport  InitialOutput=0
  tag scope: I_DCDC=global
  wires:
  Transfer Fcn (with initial outputs)2/1 -> Current controller DISCRETE1/1(ifc), Mux/2
  Duty Cycles/1(dc) -> Duty cycle/1
  Current controller DISCRETE1/1(Ec) -> Duty Cycles/1(Ec)
  Zero-Order Hold1/1 -> Transfer Fcn (with initial outputs)2/1
  iref/1 -> Fuel cell current limit/1
  ifc/1 -> Zero-Order Hold1/1
  Fuel cell current limit/1 -> Current controller DISCRETE1/2(iref), Mux/1
  Mux/1 -> [I_DCDC]

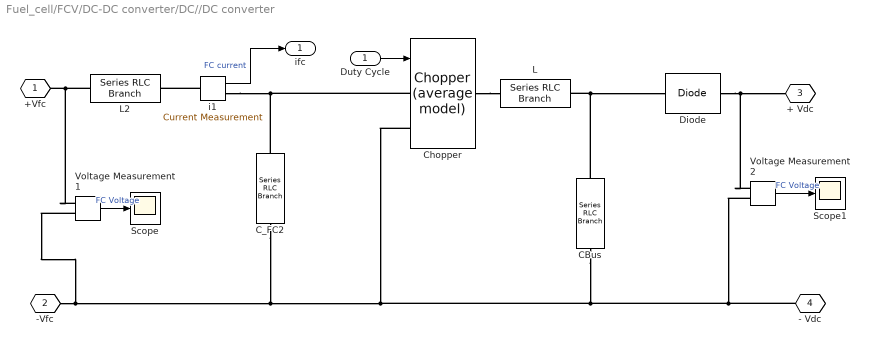
== system Fuel_cell/FCV/DC-DC converter/DC//DC converter ==
  Duty Cycle : Inport
  CBus : powerlib/Elements/Series RLC Branch  LConnTagsString=__new0  RConnTagsString=__new0  BranchType=RC  Resistance=0.2  Inductance=1e-3  SetiL0=off  InitialCurrent=0  Capacitance=1000e-6  Setx0=on  InitialVoltage=200  Measurements=None
  C_FC2 : powerlib/Elements/Series RLC Branch  LConnTagsString=__new0  RConnTagsString=__new0  BranchType=RC  Resistance=0.2  Inductance=1e-3  SetiL0=off  InitialCurrent=0  Capacitance=1000e-6  Setx0=on  InitialVoltage=420  Measurements=None
  Chopper : DC6DriveInternalModels/Chopper (average model)  SnubberResistance=10e3  SnubberCapacitance=inf  Ron=1e-3  ForwardVoltages=[1.3,1.3]  IGBTParameters=[0,0]  converterType=Inverter
      settings: SourceProductBaseCode=PS
  Diode : powerlib/Power Electronics/Diode  Ron=0.001  Lon=0  Vf=0  IC=0  UseSnubber=off  Rs=1e4  Cs=inf  Measurements=off
  L : powerlib/Elements/Series RLC Branch  LConnTagsString=__new0  RConnTagsString=__new0  BranchType=L  Resistance=0.3  Inductance=500e-6  SetiL0=off  InitialCurrent=0  Capacitance=100e-6  Setx0=off  InitialVoltage=0  Measurements=None
  L2 : powerlib/Elements/Series RLC Branch  LConnTagsString=__new0  RConnTagsString=__new0  BranchType=L  Resistance=1  Inductance=1000e-6  SetiL0=on  InitialCurrent=0  Capacitance=100e-6  Setx0=off  InitialVoltage=0  Measurements=None
  Scope : Scope
  Scope1 : Scope
  Voltage Measurement1 : powerlib/Measurements/Voltage Measurement  PhasorSimulation=off  OutputType=Complex  PSBequivalent=0
  Voltage Measurement2 : powerlib/Measurements/Voltage Measurement  PhasorSimulation=off  OutputType=Complex  PSBequivalent=0
  i1 : powerlib/Measurements/Current Measurement  PhasorSimulation=off  OutputType=Complex  PSBequivalent=0
  +Vfc : PMIOPort  Tag=PMCPort  Side=Left
  -Vfc : PMIOPort  Tag=PMCPort  Port=2  Side=Left
  + Vdc : PMIOPort  Tag=PMCPort  Port=3  Side=Right
  - Vdc : PMIOPort  Tag=PMCPort  Port=4  Side=Right
  ifc : Outport
  wires:
  Duty Cycle/1 -> Chopper/1
  i1/1 -> ifc/1  "FC current"
  Voltage Measurement1/1 -> Scope/1  "FC Voltage"
  Voltage Measurement2/1 -> Scope1/1  "FC Voltage"
  connections:
  L2/LConn1 -- Voltage Measurement1/LConn1 -- +Vfc/RConn1
  Chopper/RConn1 -- L/RConn1
  -Vfc/RConn1 -- Voltage Measurement1/LConn2 -- Voltage Measurement2/LConn2 -- - Vdc/RConn1 -- CBus/RConn1 -- Chopper/LConn2 -- C_FC2/RConn1
  CBus/LConn1 -- L/LConn1 -- Diode/LConn1
  i1/LConn1 -- L2/RConn1
  Diode/RConn1 -- Voltage Measurement2/LConn1 -- + Vdc/RConn1
  Chopper/LConn1 -- i1/RConn1 -- C_FC2/LConn1

== system Fuel_cell/FCV/Subsystem1/Measures ==
  Current Measurement : powerlib/Measurements/Current Measurement  Tag=PoWeRsYsTeMmEaSuReMeNt  PhasorSimulation=off  OutputType=Magnitude  PSBequivalent=0
  Current Measurement1 : powerlib/Measurements/Current Measurement  Tag=PoWeRsYsTeMmEaSuReMeNt  PhasorSimulation=off  OutputType=Magnitude  PSBequivalent=0
  Current Measurement2 : powerlib/Measurements/Current Measurement  Tag=PoWeRsYsTeMmEaSuReMeNt  PhasorSimulation=off  OutputType=Magnitude  PSBequivalent=0
  Mux1 : Mux  Inputs=3
  Ta : PMIOPort  Side=Left
  Tb : PMIOPort  Port=2  Side=Left
  Tc : PMIOPort  Port=3  Side=Left
  Mta : PMIOPort  Port=4  Side=Right
  Mtb : PMIOPort  Port=5  Side=Right
  Mtc : PMIOPort  Port=6  Side=Right
  I_abc : Outport
  wires:
  Mux1/1 -> I_abc/1
  Current Measurement2/1 -> Mux1/3
  Current Measurement/1 -> Mux1/1
  Current Measurement1/1 -> Mux1/2
  connections:
  Current Measurement2/RConn1 -- Mtc/RConn1
  Tc/RConn1 -- Current Measurement2/LConn1
  Ta/RConn1 -- Current Measurement/LConn1
  Current Measurement/RConn1 -- Mta/RConn1
  Tb/RConn1 -- Current Measurement1/LConn1
  Current Measurement1/RConn1 -- Mtb/RConn1
